simulink model "Fahrzeugmodell_Sprungantwort"  (R2014a)
settings: Solver=ode45  StartTime=0.0  StopTime=10.0  MaxStep=1e-3  RelTol=1e-3
InitFcn:
  | Fahrzeugmodell_Parameter;
undefined symbols (not defined in the file): c, d, l0, mA, y0
libraries: simulink x1
settings Model: Creator=Glöckler  LastModifiedBy=Glöckler
settings DataIOCC: SignalLoggingSaveFormat=ModelDataLogs
settings OptimizationCC: ExpressionDepthLimit=2147483647
settings DebuggingCC: UnderspecifiedInitializationDetection=Classic  FcnCallInpInsideContextMsg=UseLocalSettings  StateNameClashWarn=warning
settings GRTTargetCC: CombineOutputUpdateFcns=off  GRTInterface=on

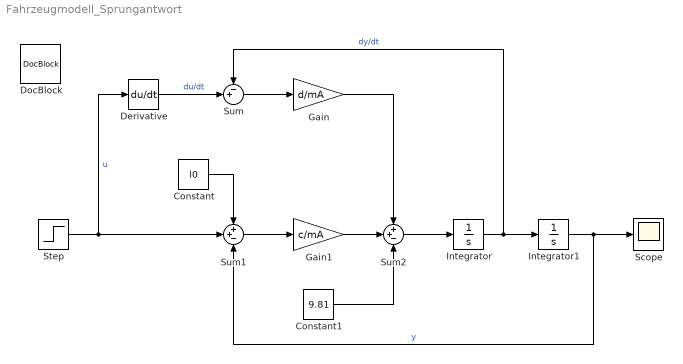
== system Fahrzeugmodell_Sprungantwort ==
  Constant : Constant  Value=l0
  Constant1 : Constant  Value=9.81
  Derivative : Derivative
  DocBlock : simulink/Model-Wide Utilities/DocBlock  DocumentType=Text
      content=|
      | Simulink-Modell des Fahrzeugmodells,
      |
      | Das Fahrzeug wird hier durch einen Sprung nach 4s angeregt;
      | Eingangsgröße x und Ausgangsgröße y werden im Scope angezeigt.
      |
      | Anfangswert y(0) = y0 steht im Block Integrator1
      |
      | Die Parameter werden automatisch geladen, siehe:
      | File/Model Properties/Callbacks/InitFcn
  Gain : Gain  Gain=d/mA
  Gain1 : Gain  Gain=c/mA
  Integrator : Integrator
  Integrator1 : Integrator  InitialCondition=y0
  Scope : Scope
      settings: TimeRange=10  YMin=0.25  YMax=0.45
  Step : Step  Time=5  After=0.1  SampleTime=0
  Sum : Sum  Inputs=-+|
  Sum1 : Sum  Inputs=++-
  Sum2 : Sum  Inputs=++-
  wires:
  Derivative/1 -> Sum/2  "du/dt"
  Step/1 -> Derivative/1, Sum1/2  "u"
  Constant/1 -> Sum1/1
  Sum/1 -> Gain/1
  Sum1/1 -> Gain1/1
  Gain1/1 -> Sum2/2
  Gain/1 -> Sum2/1
  Constant1/1 -> Sum2/3
  Sum2/1 -> Integrator/1
  Integrator/1 -> Integrator1/1, Sum/1  "dy/dt"
  Integrator1/1 -> Sum1/3, Scope/1  "y"
